simulink model "PANCs_matlabfunction"  (R2020a)
settings: Solver=ode3  StartTime=0.0  StopTime=10.0  FixedStep=0.1  RelTol=1e-3  EnableMultiTasking=on
settings Model: Creator=CARVALHO  LastModifiedBy=Arnaldo
settings DataIOCC: LimitDataPoints=on  SaveFormat=Array  ReturnWorkspaceOutputs=off
settings OptimizationCC: LifeSpan=inf
settings DebuggingCC: SFUnexpectedBacktrackingDiag=warning  SFNoUnconditionalDefaultTransitionDiag=warning  SFExecutionAtInitializationDiag=none  ArithmeticOperatorsInVariantConditions=warning
settings HardwareCC: ProdBitPerPointer=32  ProdBitPerSizeT=32  ProdBitPerPtrDiffT=32  ProdLargestAtomicFloat=None  ProdIntDivRoundTo=Undefined  ProdEndianess=Unspecified  ProdWordSize=32  ProdHWDeviceType=32-bit Generic
settings ModelReferenceCC: PropagateSignalLabelsOutOfModel=off
settings SFSimCC: SimUseLocalCustomCode=off  CustomCodeUndefinedFunction=UseInterfaceOnly
settings RTWCC: RTWUseLocalCustomCode=off
settings CodeAppCC: StateflowObjectComments=on
settings GRTTargetCC: TargetLangStandard=C89/C90 (ANSI)
settings ConfigComp: CovMetricSettings=dw  CovHtmlReporting=on  CovSaveCumulativeToWorkspaceVar=on  CovSaveSingleToWorkspaceVar=on  CovExternalEMLEnable=off

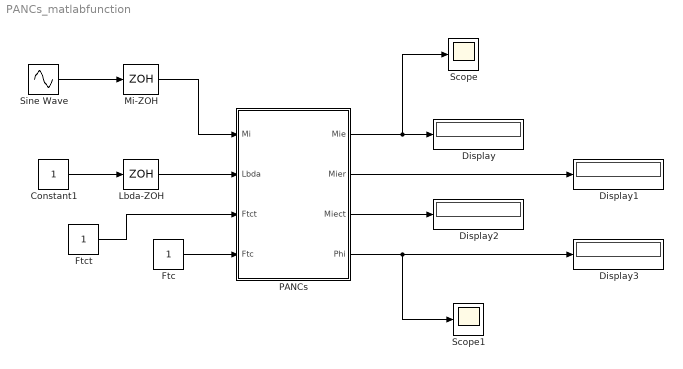
== system PANCs_matlabfunction ==
  Constant1 : Constant
  Display{,1..3} (4 alike) : Display
  Ftc : Constant
  Ftct : Constant
  Lbda-ZOH : ZeroOrderHold  SampleTime=0.1
  Mi-ZOH : ZeroOrderHold  SampleTime=0.1
  PANCs : MATLAB Function  TreatAsAtomicUnit=on
  Scope : Scope
  Scope1 : Scope
  Sine Wave : Sin  Amplitude=0.3  Bias=0.5
  wires:
  Mi-ZOH/1 -> PANCs/1(Mi)
  Lbda-ZOH/1 -> PANCs/2(Lbda)
  Constant1/1 -> Lbda-ZOH/1
  PANCs/1(Mie) -> Scope/1, Display/1
  PANCs/2(Mier) -> Display1/1
  PANCs/3(Miect) -> Display2/1
  PANCs/4(Phi) -> Scope1/1, Display3/1
  Ftc/1 -> PANCs/4(Ftc)
  Ftct/1 -> PANCs/3(Ftct)
  Sine Wave/1 -> Mi-ZOH/1

== matlab function PANCs_matlabfunction/PANCs ==
  data: Mi input; Mie output; Lbda input; Mier output; Miect output; Phi output; Ftct input; Ftc input
function [Mie,Mier, Miect, Phi] = fcn(Mi, Lbda, Ftct, Ftc)
% Módulo NAP e cNAP completo, com ajustes FtC, FtCt
% Ajustar Tempo de Amostragens dos ZOH aplicados à entrada da cNAP
if Mi>1 %Limite entre 0 e 1 para Mi
  Mi_input = 1;
elseif (Mi>=0)&&(Mi<=1)
  Mi_input = Mi;
else
  Mi_input = 0;
end
if Lbda>1 %Limite entre 0 e 1 para Lbda
  Lbda_input = 1;
elseif (Lbda>=0)&&(Lbda<=1)
  Lbda_input = Lbda;
else
  Lbda_input = 0;
end
if Ftc>1 %Limite entre 0 e 1 para Ftc
  Ftc_input = 1;
elseif (Ftc>=0)&&(Ftc<=1)
  Ftc_input = Ftc;
else
  Ftc_input = 0;
end
if Ftct>1 %Limite entre 0 e 1 para Ftct
  Ftct_input = 1;
elseif (Ftct>=0)&&(Ftct<=1)
  Ftct_input = Ftct;
else
  Ftct_input = 0;
end
Vscc=(1+Ftc_input)/2;Vicc=(1-Ftc_input)/2; %Limites superior Vscc e inferior Vicc
Vscct=(1+Ftct_input)/2;Vicct=(1-Ftct_input)/2; %Limites superior Vscct e inferior Vicct
GC=Mi_input-Lbda_input;
GCT=Mi_input+Lbda_input-1;
Mie=(GC+1)/2;
Phi=1-abs(GCT);
D=((1-abs(GC))^2+GCT^2)^0.5;
if GC>0
      GCR=1-D;
elseif GC<0
       GCR=D-1;
  else
      GCR=0;
  end
Mier=(GCR+1)/2;
Miect=(GCT+1)/2;
     if GCT>0
         Phi=+abs(Phi);
     elseif GCT<0
         Phi=-abs(Phi);
     else
         Phi=1;
     end 
     if Miect>=Vicct && Miect<=Vscct
         if Mier<=Vscc && Mier >= Vicc
         Mie=Mie;
         Mier=Mier;
     else
         Mie=0.5;
         Mier=0.5;
         end
     else
         Miect=0.5;
     end
end
